simulink model "sysgenConcatenatedFEC"  (Simulink 7.4)
settings: Solver=ode45  SolverMode=SingleTasking  StartTime=0.0  StopTime=5000  RelTol=1e-3
undefined symbols (not defined in the file or in its folder): De, Interleaver, interleaver
libraries: xbsIndex_r4 x119, commchan3 x2, commdigbbndpm3 x2, xbsCopyrightNotice_r4 x1
(part 1 of 2)
settings Model: Creator=alexc  LastModifiedBy=douangp
settings DataIOCC: SignalLoggingName=sigsOut
settings OptimizationCC: BlockReduction=off  BooleanDataType=off  InlineInvariantSignals=on  InitFltsAndDblsToZero=on
settings DebuggingCC: SaveWithParameterizedLinksMsg=none  SignalResolutionControl=TryResolveAllWithWarning  SolverPrmCheckMsg=none  MultiTaskDSMMsg=warning  MultiTaskCondExecSysMsg=none  StrictBusMsg=None
settings HardwareCC: TargetUnknown=on
settings RTWCC: IncludeERTFirstTime=on
settings GRTTargetCC: TargetFcnLib=ansi_tfl_tmw.mat

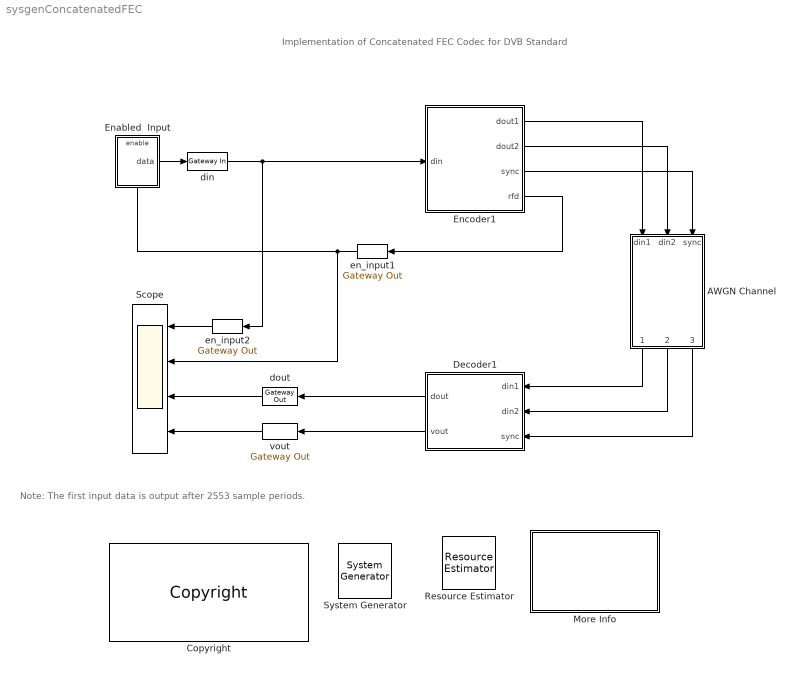
== system sysgenConcatenatedFEC ==
  note: Implementation of Concatenated
      | FEC Codec for DVB Standard
  note: Note: The first input data is output after 2553 sample periods.
  " System Generator" : xbsIndex_r4/ System Generator  Tag=genX  SystemSampleTime=-1  xilinxfamily=virtex6  part=xc6vlx240t  speed=-1  package=ff1156  synthesis_tool=XST  clock_wrapper=Clock Enables  directory=./netlist  testbench=off  simulink_period=1/8  sysclk_period=5  dcm_input_clock_period=100  incr_netlist=off  trim_vbits=Everywhere in SubSystem  dbl_ovrd=According to Block Masks  core_generation=According to Block Masks  run_coregen=off  deprecated_control=off  eval_field=0  block_type=sysgen
      settings: block_version=9.2.00
  AWGN Channel : Subsystem  mask{snr=4}
  Copyright : xbsCopyrightNotice_r4/Copyright  copyrighttext="Copyright (c) 2010  by  Xilinx, Inc. All rights reserved.<br><br>This file contains proprietary, confidential information of Xilinx, Inc., is distributed under licensefrom Xilinx, Inc., and may be used, copied and/or disclosed only pursuant to the terms of a valid licenseagreement with Xilinx, Inc. Xilinx hereby grants you a license to use this file solely for design,simulation, implementation and creation of design files limited to Xilinx devices or technologies. Use with non-Xilinx devices or technologies is expressly prohibited and immediately terminates your license unless covered by a separate agreement.<br><br>Xilinx is providing this design, code, or information \"as-is\" solely for use in developing programs and solutions for Xilinx devices, with no obligation on the part of Xilinx to provide support. By providingthis design, code, or information as one possible implementation of this feature, application or standard,Xilinx is making no representation that this implementation is free from any claims of infringement. Youare responsible for obtaining any rights you may require for your implementation. Xilinx expressly disclaimsany warranty whatsoever with respect to the adequacy of the implementation, including but not limited to anywarranties or representations that this implementation is free from claims of infringement, implied warrantiesof merchantability or fitness for a particular purpose.<br><br>Xilinx products are not intended for use in life support appliances, devices, or systems. Use in such applications is expressly prohibited.<br><br>Any modifications that are made to the Source Code are done at the user's sole risk and will be unsupported.<br><br>This copyright and support notice must be retained as part of this text at all times. (c) Copyright 1995-2010 Xilinx, Inc. All rights reserved."  block_type=copyright
      settings: block_version=10.1.00
      settings: infoedit=|
      | Copyright(C) 2008 by  Xilinx, Inc. All rights reserved.<br>
      | <br>
      | This file contains proprietary, confidential information of Xilinx, Inc., is distributed under license
      | from Xilinx, Inc., and may be used, copied and/or disclosed only pursuant to the terms of a valid license
      | agreement with Xilinx, Inc. Xilinx hereby grants you a license to use this file solely for design,
      | simulation, implementation and creation of design files limited to Xilinx devices or technologies. Use
      | with non-Xilinx devices or technologies is expressly prohibited and immediately terminates your license
      | unless covered by a separate agreement.<br>
      | <br>
      | Xilinx is providing this design, code, or information "as-is" solely for use in developing programs and
      | solutions for Xilinx devices, with no obligation on the part of Xilinx to provide support. By providing
      | this design, code, or information as one possible implementation of this feature, application or standard,
      | Xilinx is making no representation that this implementation is free from any claims of infringement. You
      | are responsible for obtaining any rights you may require for your implementation. Xilinx expressly disclaims
      | any warranty whatsoever with respect to the adequacy of the implementation, including but not limited to any
      | warranties or representations that this implementation is free from claims of infringement, implied warranties
      | of merchantability or fitness for a particular purpose.<br>
      | <br>
      | Xilinx products are not intended for use in life support appliances, devices, or systems. Use in such
      | applications is expressly prohibited.<br>
      | <br>
      | Any modifications that are made to the Source Code are done at the user's sole risk and will be unsupported.<br>
      | <br>
      | This copyright and support notice must be retained as part of this text at all times.
      | (c) Copyright 1995-2008 Xilinx, Inc. All rights reserved.
  Decoder1 : Subsystem
  Enabled  Input : Subsystem  TreatAsAtomicUnit=on
  Encoder1 : Subsystem
  More Info : Subsystem
      mask Display: disp('Double click\n for\n more information.')
  Resource Estimator : xbsIndex_r4/Resource Estimator  Tag=resEstTag  Slices=2727  FFs=2644  BRAMs=8  LUTs=4673  IOBs=27  EBMs=0  TBUFs=0  xl_use_estimator_area=off  est_options=Estimate  xl_estimator_area=[2727 2644 8 4673 27 0 0]  mrp_directory=./sysgenConcatenatedFEC_work  simulink_period=1/8  block_type=resource_estimator
      settings: AttributesFormatString=Resource\nEstimator  block_version=9.2.00
  Scope : Scope  NumInputPorts=4
      settings: TimeRange=5000  YMin=-1~0~-1~0  YMax=0.75~1~1~1  MaxDataPoints=30000
  din : xbsIndex_r4/Gateway In  arith_type="Signed  (2's comp)"  n_bits=8  bin_pt=6  quantization="Round  (unbiased: +/- Inf)"  overflow=Saturate  period=1  dbl_ovrd=off  timing_constraint=None  locs_specified=off  LOCs={}  hdl_port=on  block_type=gatewayin
      settings: infoedit="Gateway in block.  Converts inputs of type Simulink integer, double and fixed point to  Xilinx fixed point type.<P><P>Hardware notes:  In hardware these blocks become top level input ports."  xl_area=[0 0 0 0 8 0 0]  block_version=VER_STRING_GOES_HERE
  dout : xbsIndex_r4/Gateway Out  hdl_port=on  timing_constraint=None  locs_specified=off  LOCs={}  block_type=gatewayout
      settings: infoedit="Gateway out block.  Converts Xilinx fixed point inputs into ouputs of type Simulink integer, double, or fixed point.<P><P>Hardware notes:  In hardware these blocks become top level output ports or are discarded, depending on how they are configured."  xl_area=[0 0 0 0 8 0 0]  block_version=VER_STRING_GOES_HERE
  en_input1 : xbsIndex_r4/Gateway Out  hdl_port=off  timing_constraint=None  locs_specified=off  LOCs={}  block_type=gatewayout
      settings: infoedit="Gateway out block.  Converts Xilinx fixed point inputs into ouputs of type Simulink integer, double, or fixed point.<br><br>Hardware notes:  In hardware these blocks become top level output ports or are discarded, depending on how they are configured."  block_version=11.4
  en_input2 : xbsIndex_r4/Gateway Out  hdl_port=off  timing_constraint=None  locs_specified=off  LOCs={}  block_type=gatewayout
      settings: infoedit="Gateway out block.  Converts Xilinx fixed point inputs into ouputs of type Simulink integer, double, or fixed point.<br><br>Hardware notes:  In hardware these blocks become top level output ports or are discarded, depending on how they are configured."  block_version=11.4
  vout : xbsIndex_r4/Gateway Out  hdl_port=on  timing_constraint=None  locs_specified=off  LOCs={}  block_type=gatewayout
      settings: infoedit="Gateway out block.  Converts Xilinx fixed point inputs into ouputs of type Simulink integer, double, or fixed point.<P><P>Hardware notes:  In hardware these blocks become top level output ports or are discarded, depending on how they are configured."  xl_area=[0 0 0 0 0 0 0]  block_version=VER_STRING_GOES_HERE
  wires:
  Decoder1/1(dout) -> dout/1
  Encoder1/4(rfd) -> en_input1/1
  Enabled  Input/1(data) -> din/1
  din/1 -> en_input2/1, Encoder1/1(din)
  AWGN Channel/1(dout1) -> Decoder1/1(din1)
  AWGN Channel/2(dout2) -> Decoder1/2(din2)
  AWGN Channel/3(sync1) -> Decoder1/3(sync)
  Encoder1/3(sync) -> AWGN Channel/3(sync)
  Encoder1/1(dout1) -> AWGN Channel/1(din1)
  Encoder1/2(dout2) -> AWGN Channel/2(din2)
  Decoder1/2(vout) -> vout/1
  dout/1 -> Scope/3
  vout/1 -> Scope/4
  en_input1/1 -> Scope/2, Enabled  Input/Enable
  en_input2/1 -> Scope/1

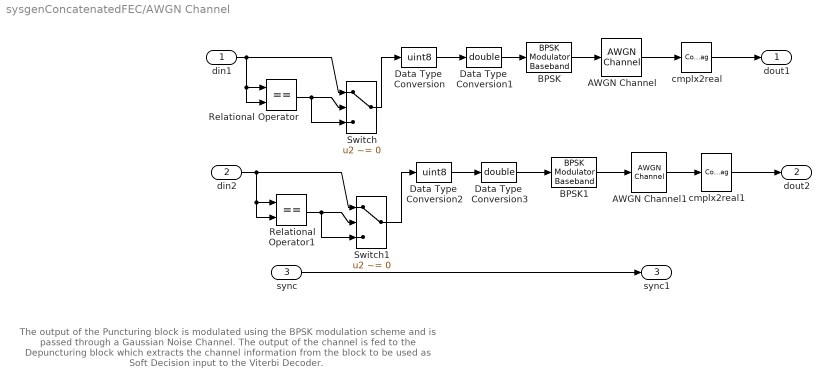
== system sysgenConcatenatedFEC/AWGN Channel ==
  note: The output of the Puncturing block is modulated using the BPSK modulation scheme and  is passed through
      | a Gaussian Noise Channel. The output of the channel is fed to the Depuncturing block which extracts the
      | channel information from the block to be used as Soft Decision input to the Viterbi Decoder.
  din1 : Inport  OutDataType=sfix(16)  OutScaling=2^0
  din2 : Inport  Port=2  OutDataType=sfix(16)  OutScaling=2^0
  sync : Inport  Port=3  OutDataType=sfix(16)  OutScaling=2^0
  AWGN Channel : commchan3/AWGN Channel  SystemSampleTime=-1  seed=54321  noiseMode="Signal to noise ratio  (SNR)"  EbNodB=10  EsNodB=10  SNRdB=snr  bitsPerSym=1  Ps=1  Tsym=1  variance=1
  AWGN Channel1 : commchan3/AWGN Channel  SystemSampleTime=-1  seed=54321  noiseMode="Signal to noise ratio  (SNR)"  EbNodB=10  EsNodB=10  SNRdB=snr  bitsPerSym=1  Ps=1  Tsym=1  variance=1
  BPSK : commdigbbndpm3/BPSK Modulator Baseband  DialogController=commDDGCreate  DialogControllerArgs=DataTag1  SystemSampleTime=-1  Ph=0  outDtype=double  outWordLen=16  outUDDataType=sfix(16)  outFracLenMode=Best precision  outFracLen=15
      link override M-PSK Modulator Baseband: outDtype=double  outFracLenMode=Best precision
  BPSK1 : commdigbbndpm3/BPSK Modulator Baseband  DialogController=commDDGCreate  DialogControllerArgs=DataTag2  SystemSampleTime=-1  Ph=0  outDtype=double  outWordLen=16  outUDDataType=sfix(16)  outFracLenMode=Best precision  outFracLen=15
  Data Type  Conversion : DataTypeConversion  OutDataTypeMode=uint8  OutDataType=sfix(16)  OutScaling=2^0  OutDataTypeStr=uint8  SaturateOnIntegerOverflow=on  RndMeth=Zero
  Data Type  Conversion1 : DataTypeConversion  OutDataTypeMode=double  OutDataType=sfix(16)  OutScaling=2^0  OutDataTypeStr=double  SaturateOnIntegerOverflow=on  RndMeth=Zero
  Data Type  Conversion2 : DataTypeConversion  OutDataTypeMode=uint8  OutDataType=sfix(16)  OutScaling=2^0  OutDataTypeStr=uint8  SaturateOnIntegerOverflow=on  RndMeth=Zero
  Data Type  Conversion3 : DataTypeConversion  OutDataTypeMode=double  OutDataType=sfix(16)  OutScaling=2^0  OutDataTypeStr=double  SaturateOnIntegerOverflow=on  RndMeth=Zero
  Relational Operator : RelationalOperator  Operator===  LogicOutDataTypeMode=boolean  OutDataTypeStr=boolean
  Relational Operator1 : RelationalOperator  Operator===  LogicOutDataTypeMode=boolean  OutDataTypeStr=boolean
  Switch : Switch  Criteria=u2 ~= 0
  Switch1 : Switch  Criteria=u2 ~= 0
  cmplx2real : ComplexToRealImag  Output=Real
  cmplx2real1 : ComplexToRealImag  Output=Real
  dout1 : Outport  OutDataType=sfix(16)  OutScaling=2^0
  dout2 : Outport  Port=2  OutDataType=sfix(16)  OutScaling=2^0
  sync1 : Outport  Port=3  OutDataType=sfix(16)  OutScaling=2^0
  wires:
  BPSK/1 -> AWGN Channel/1
  BPSK1/1 -> AWGN Channel1/1
  AWGN Channel/1 -> cmplx2real/1
  AWGN Channel1/1 -> cmplx2real1/1
  cmplx2real/1 -> dout1/1
  cmplx2real1/1 -> dout2/1
  sync/1 -> sync1/1
  Data Type  Conversion3/1 -> BPSK1/1
  Data Type  Conversion1/1 -> BPSK/1
  Data Type  Conversion/1 -> Data Type  Conversion1/1
  Data Type  Conversion2/1 -> Data Type  Conversion3/1
  din1/1 -> Relational Operator/1, Relational Operator/2, Switch/1
  Relational Operator/1 -> Switch/2, Switch/3
  Switch/1 -> Data Type  Conversion/1
  din2/1 -> Relational Operator1/1, Relational Operator1/2, Switch1/1
  Relational Operator1/1 -> Switch1/2, Switch1/3
  Switch1/1 -> Data Type  Conversion2/1

== system sysgenConcatenatedFEC/Decoder1 ==
  note: Depuncturing
  note: Inner
      | Decoder
  note: Convolutional
      | Deinterleaver
  note: Outer
      | Decoder
  note: Concatenated Decoder
  din1 : Inport  OutDataType=sfix(16)  OutScaling=2^0
  din2 : Inport  Port=2  OutDataType=sfix(16)  OutScaling=2^0
  sync : Inport  Port=3  OutDataType=sfix(16)  OutScaling=2^0
  cvdeint : Subsystem
  depunc : Subsystem
  rsdec : Subsystem
  vitdec : Subsystem
  dout : Outport  OutDataType=sfix(16)  OutScaling=2^0
  vout : Outport  Port=2  OutDataType=sfix(16)  OutScaling=2^0
  wires:
  rsdec/2(data1) -> vout/1
  rsdec/1(data) -> dout/1
  sync/1 -> depunc/3(sync)
  din2/1 -> depunc/2(din2)
  din1/1 -> depunc/1(din1)
  cvdeint/2(vout) -> rsdec/2(vin)
  vitdec/2(vout) -> cvdeint/2(vin)
  depunc/3(vin) -> vitdec/3(vin)
  cvdeint/1(dout) -> rsdec/1(din)
  vitdec/1(dout) -> cvdeint/1(din)
  depunc/2(dout2) -> vitdec/2(din2)
  depunc/1(dout1) -> vitdec/1(din1)

== system sysgenConcatenatedFEC/Enabled  Input ==
  note: The input to the concatenated coder is a sine wave which is enabled using the RFD (Ready for Data)
      | output of the Outer Encoder.
  Enable : EnablePort  PropagateVarSize=During execution
  Sine Wave : Sin  SineType=Sample based  Amplitude=1  Bias=0  Frequency=1  Phase=0  Samples=60  SampleTime=1  Offset=0
  data : Outport  OutDataType=sfix(16)  OutScaling=2^0
  wires:
  Sine Wave/1 -> data/1

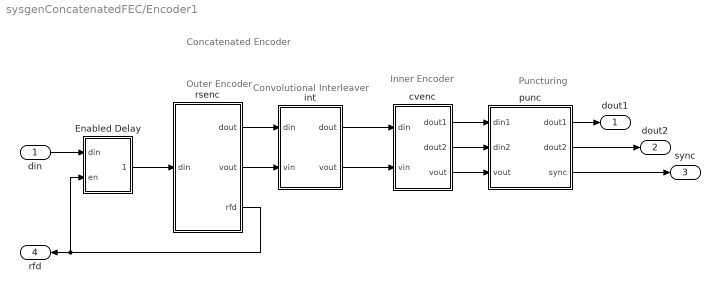
== system sysgenConcatenatedFEC/Encoder1 ==
  note: Outer
      | Encoder
  note: Convolutional
      | Interleaver
  note: Inner
      | Encoder
  note: Puncturing
  note: Concatenated Encoder
  din : Inport  OutDataType=sfix(16)  OutScaling=2^0
  Enabled Delay : Subsystem
  cvenc : Subsystem
  int : Subsystem
  punc : Subsystem
  rsenc : Subsystem
  dout1 : Outport  OutDataType=sfix(16)  OutScaling=2^0
  dout2 : Outport  Port=2  OutDataType=sfix(16)  OutScaling=2^0
  sync : Outport  Port=3  OutDataType=sfix(16)  OutScaling=2^0
  rfd : Outport  Port=4  OutDataType=sfix(16)  OutScaling=2^0
  wires:
  Enabled Delay/1(dout) -> rsenc/1(din)
  din/1 -> Enabled Delay/1(din)
  rsenc/1(dout) -> int/1(din)
  int/1(dout) -> cvenc/1(din)
  rsenc/2(vout) -> int/2(vin)
  int/2(vout) -> cvenc/2(vin)
  cvenc/3(vout) -> punc/3(vout)
  cvenc/2(dout2) -> punc/2(din2)
  cvenc/1(dout1) -> punc/1(din1)
  punc/3(sync) -> sync/1
  punc/2(dout2) -> dout2/1
  punc/1(dout1) -> dout1/1
  rsenc/3(rfd) -> Enabled Delay/2(en), rfd/1

== system sysgenConcatenatedFEC/More Info ==
  note: This design demonstrates a concatenated forward error correction scheme using the
      |  blocks provided in the Xilinx Communication library. The scheme is implemented
      | according to the specifications provided in the European Telecommunication Standard
      | (ETS 300 421) for Digital Video Broadcasting.
  note: Implementation of Concatenated FEC Codec for DVB Standard

== system sysgenConcatenatedFEC/Decoder1/cvdeint ==
  note: The Convolutional Deinterleaver specified in the standard is implemented by selecting Deinterleaver mode in the
      | Interleaver Deinterleaver block in the Xilinx Communication library. The Deinterleaver has 12 branches with the
      | constant difference between branch lengths being 17 shift registers. The convolutional deinterleaving is based on
      | the Forney type architecture. The Deinterleaver block synchronizes its output to the first valid data received at the input.
      | The Delay block at the input of the deinterleaver is used for pipelining the design.
      |
      | A single pulse is required at the "fd" (First Data) input and it has to be lined up with the "nd" (New Data) signal.
      | To accomplish this,  a simple single-shot circuit is used (Rising Edge Detector) to detect a low-to-high transition from "vin".
  din : Inport  OutDataType=sfix(16)  OutScaling=2^0
  vin : Inport  Port=2  OutDataType=sfix(16)  OutScaling=2^0
  Delay : xbsIndex_r4/Delay  en=off  latency=1  dbl_ovrd=off  reg_retiming=off  block_type=delay
      settings: infoedit="Delay line having  configurable length.<P><P>Hardware notes: A delay line is a chain, each link of which is an SRL16 followed by a flip-flop. If register retiming is enabled, the delay line is a chain of flip-flops."  xl_area=[0, 0, 0, 0, 0, 0, 0]  block_version=VER_STRING_GOES_HERE
  Delay1 : xbsIndex_r4/Delay  en=off  latency=1  dbl_ovrd=off  reg_retiming=off  block_type=delay
      settings: infoedit="Delay line having  configurable length.<P><P>Hardware notes: A delay line is a chain, each link of which is an SRL16 followed by a flip-flop. If register retiming is enabled, the delay line is a chain of flip-flops."  xl_area=[0, 0, 0, 0, 0, 0, 0]  block_version=VER_STRING_GOES_HERE
  "Interleaver/De-interleaver 6.0 " : xbsIndex_r4/Interleaver//De-interleaver 6.0   memory_style=Automatic  symbol_width=8  sid_type=Forney  mode=Deinterleaver  symbol_memory=Internal  number_of_branches=12  architecture=ROM_based  number_of_configurations=1  branch_length_constant=17  branch_length_coe_file_name='no_coe_file_loaded'  branch_length_type=constant_difference_between_consecutive_branches  number_of_rows_constant_value=15  row_port_width=4  minimum_rows=15  number_of_rows_selectable_value=4  number_of_rows=constant  number_of_columns_constant_value=15  col_port_width=4  minimum_columns=15  number_of_columns_selectable_value=4  number_of_columns=constant  row_permutations=None  column_permutations=None  coe_file='no_coe_file_loaded'  block_size_constant_value=225  block_size_port_width=8  block_size_type=rows_columns  row_valid=off  block_size_valid=off  ce=off  rfd=off  row_sel_valid=off  block_start=off  sclr=off  rffd=off  col_valid=off  block_end=off  ndo=off  fdo=off  col_sel_valid=off  nd=on  rdy=on  pipelining=minimum  ip_name=Interleaver/De-interleaver  ip_version=6.0  dsptool_ready=true  ipcore_usecache=true  ipcore_useipmodelcache=true  wrapper_available=true  port_translation_map={ 'ce' => 'en', 'sclr' => 'rst'}  structural_sim=false  ipcore_verbose=false  ipcore_do_not_force_period=true  block_type=sid_v6_0
      settings: infoedit=Forney Information : The Forney type is composed of a user-defined number of delay-line shift registers. The length of each of the delay-line shift registers can be specified using a COE file, or by setting the difference in the length of consecutive delay line shift registers to a fixed, user-defined value. <br> Rectangular Information : The Rectangular Block type is composed of a rectangular array of memory elements, where the number of rows and columns in the array is user-defined. The number of rows and columns can be constant or run-time configurable. The elements are written to row-wise, and read out column-wise, or vice versa, depending on which mode is selected. This type supports user-defined inter-row and inter-column permutations. It also supports pruning - cases where the block size is less than the product of the number of rows and columns.  block_version=12.1
  Rising Edge Detector1 : Subsystem
  dout : Outport  OutDataType=sfix(16)  OutScaling=2^0
  vout : Outport  Port=2  OutDataType=sfix(16)  OutScaling=2^0
  wires:
  "Interleaver/De-interleaver 6.0 "/2 -> vout/1
  vin/1 -> Rising Edge Detector1/1(Din), Delay1/1
  din/1 -> Delay/1
  "Interleaver/De-interleaver 6.0 "/1 -> dout/1
  Delay/1 -> "Interleaver/De-interleaver 6.0 "/1
  Delay1/1 -> "Interleaver/De-interleaver 6.0 "/2
  Rising Edge Detector1/1(Dout) -> "Interleaver/De-interleaver 6.0 "/3

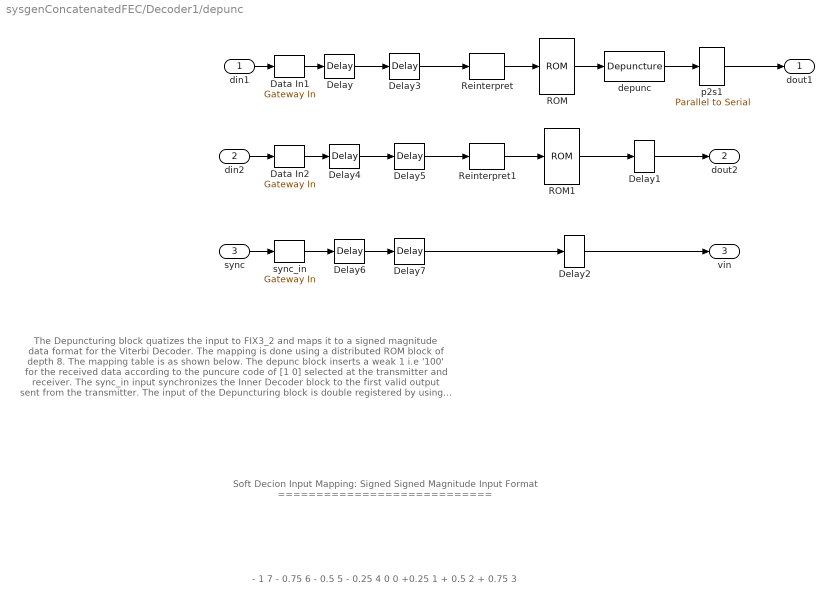
== system sysgenConcatenatedFEC/Decoder1/depunc ==
  note: Soft Decion Input Mapping:
      |
      | Signed            Signed Magnitude
      | Input                Format
      | ============================
  note: - 1                                7
      | - 0.75                                 6
      | - 0.5                                  5
      | - 0.25                                 4
      | 0                                0
      | +0.25                                 1
      | + 0.5                                  2
      | + 0.75                                 3
  note: The Depuncturing block quatizes the input to FIX3_2 and maps it to a signed magnitude data format for
      | the Viterbi Decoder. The mapping is done using a distributed ROM block of depth 8. The mapping table is
      | as shown below. The depunc block inserts a weak 1 i.e '100' for the received data according to the puncure
      | code of  [1 0] selected at the transmitter and receiver. The sync_in input synchronizes the Inner Decoder block
      | to the first valid output sent from the transmitter. The input of the Depuncturing block is double registered by using
      | the delay blocks.
  din1 : Inport  OutDataType=sfix(16)  OutScaling=2^0
  din2 : Inport  Port=2  OutDataType=sfix(16)  OutScaling=2^0
  sync : Inport  Port=3  OutDataType=sfix(16)  OutScaling=2^0
  Data In1 : xbsIndex_r4/Gateway In  arith_type="Signed  (2's comp)"  n_bits=3  bin_pt=2  quantization="Round  (unbiased: +/- Inf)"  overflow=Saturate  period=1/4  dbl_ovrd=off  timing_constraint=None  locs_specified=off  LOCs={}  hdl_port=on  block_type=gatewayin
      settings: infoedit="Gateway in block.  Converts inputs of type Simulink integer, double and fixed point to  Xilinx fixed point type.<P><P>Hardware notes:  In hardware these blocks become top level input ports."  xl_area=[0 0 0 0 3 0 0]  block_version=VER_STRING_GOES_HERE
  Data In2 : xbsIndex_r4/Gateway In  arith_type="Signed  (2's comp)"  n_bits=3  bin_pt=2  quantization="Round  (unbiased: +/- Inf)"  overflow=Saturate  period=1/8  dbl_ovrd=off  timing_constraint=None  locs_specified=off  LOCs={}  hdl_port=on  block_type=gatewayin
      settings: infoedit="Gateway in block.  Converts inputs of type Simulink integer, double and fixed point to  Xilinx fixed point type.<P><P>Hardware notes:  In hardware these blocks become top level input ports."  xl_area=[0 0 0 0 3 0 0]  block_version=VER_STRING_GOES_HERE
  Delay{,3..7} (6 alike) : xbsIndex_r4/Delay  en=off  latency=1  dbl_ovrd=off  reg_retiming=off  block_type=delay
      Delay settings: infoedit="Delay line having  configurable length.<P><P>Hardware notes: A delay line is a chain, each link of which is an SRL16 followed by a flip-flop. If register retiming is enabled, the delay line is a chain of flip-flops."  xl_area=[2 3 0 0 0 0 0]  block_version=VER_STRING_GOES_HERE
      Delay3 settings: infoedit="Delay line having  configurable length.<P><P>Hardware notes: A delay line is a chain, each link of which is an SRL16 followed by a flip-flop. If register retiming is enabled, the delay line is a chain of flip-flops."  xl_area=[2 3 0 0 0 0 0]  block_version=VER_STRING_GOES_HERE
      Delay4 settings: infoedit="Delay line having  configurable length.<P><P>Hardware notes: A delay line is a chain, each link of which is an SRL16 followed by a flip-flop. If register retiming is enabled, the delay line is a chain of flip-flops."  xl_area=[2 3 0 0 0 0 0]  block_version=VER_STRING_GOES_HERE
      Delay5 settings: infoedit="Delay line having  configurable length.<P><P>Hardware notes: A delay line is a chain, each link of which is an SRL16 followed by a flip-flop. If register retiming is enabled, the delay line is a chain of flip-flops."  xl_area=[2 3 0 0 0 0 0]  block_version=VER_STRING_GOES_HERE
      Delay6 settings: infoedit="Delay line having  configurable length.<P><P>Hardware notes: A delay line is a chain, each link of which is an SRL16 followed by a flip-flop. If register retiming is enabled, the delay line is a chain of flip-flops."  xl_area=[1 1 0 0 0 0 0]  block_version=VER_STRING_GOES_HERE
      Delay7 settings: infoedit="Delay line having  configurable length.<P><P>Hardware notes: A delay line is a chain, each link of which is an SRL16 followed by a flip-flop. If register retiming is enabled, the delay line is a chain of flip-flops."  xl_area=[1 1 0 0 0 0 0]  block_version=VER_STRING_GOES_HERE
  Delay1 : xbsIndex_r4/Delay  en=off  latency=6  dbl_ovrd=off  reg_retiming=off  block_type=delay
      settings: infoedit="Delay line having  configurable length.<P><P>Hardware notes: A delay line is a chain, each link of which is an SRL16 followed by a flip-flop. If register retiming is enabled, the delay line is a chain of flip-flops."  xl_area=[2 3 0 3 0 0 0]  block_version=VER_STRING_GOES_HERE
  Delay2 : xbsIndex_r4/Delay  en=off  latency=6  dbl_ovrd=off  reg_retiming=off  block_type=delay
      settings: infoedit="Delay line having  configurable length.<P><P>Hardware notes: A delay line is a chain, each link of which is an SRL16 followed by a flip-flop. If register retiming is enabled, the delay line is a chain of flip-flops."  xl_area=[1 1 0 1 0 0 0]  block_version=VER_STRING_GOES_HERE
  ROM : xbsIndex_r4/ROM  depth=8  initVector="[ 0  1 2 3 7 6 5 4]"  distributed_mem=Distributed memory  rst=off  init_reg=0  en=off  latency=0  arith_type=Unsigned  n_bits=3  bin_pt=0  dbl_ovrd=off  optimize=Area  use_rpm=off  block_type=sprom
      settings: xl_area=[2 0 0 3 0 0 0]  block_version=VER_STRING_GOES_HERE
  ROM1 : xbsIndex_r4/ROM  depth=8  initVector="[ 0  1 2 3 7 6 5 4]"  distributed_mem=Distributed memory  rst=off  init_reg=0  en=off  latency=0  arith_type=Unsigned  n_bits=3  bin_pt=0  dbl_ovrd=off  optimize=Area  use_rpm=off  block_type=sprom
      settings: xl_area=[2 0 0 3 0 0 0]  block_version=VER_STRING_GOES_HERE
  Reinterpret : xbsIndex_r4/Reinterpret  force_arith_type=on  arith_type=Unsigned  force_bin_pt=on  bin_pt=0  block_type=cast
      settings: infoedit="Changes type of samples without altering their binary representation.<P><P>Hardware notes: In hardware this block costs nothing.<P><P>Example:  Suppose the input is 6 bits wide, signed, with 2 fractional bits, and the output is forced to unsigned with 0 fractional bits.  Then an input of -2.0 (1110.00 in binary 2's complement) becomes an output of 56 (111000 in binary)."  block_version=VER_STRING_GOES_HERE
  Reinterpret1 : xbsIndex_r4/Reinterpret  force_arith_type=on  arith_type=Unsigned  force_bin_pt=on  bin_pt=0  block_type=cast
      settings: infoedit="Changes type of samples without altering their binary representation.<P><P>Hardware notes: In hardware this block costs nothing.<P><P>Example:  Suppose the input is 6 bits wide, signed, with 2 fractional bits, and the output is forced to unsigned with 0 fractional bits.  Then an input of -2.0 (1110.00 in binary 2's complement) becomes an output of 56 (111000 in binary)."  block_version=VER_STRING_GOES_HERE
  depunc : xbsIndex_r4/Depuncture  insert_char=[1 0]  insert_string='100'  dbl_ovrd=off  block_type=insert
      settings: infoedit="Depunctures convolutional codes.  Reads values from the input port, then inserts symbols at the locations specified by zeros in the puncture code, and presents the results at the output port. <P><P>Hardware notes: In hardware this block costs nothing."  block_version=VER_STRING_GOES_HERE
  p2s1 : xbsIndex_r4/Parallel to Serial  output_order=Least Significant Word First  arith_type=Unsigned  output_bits=3  bin_pt=0  en=off  latency=0  dbl_ovrd=off  block_type=p2s
      settings: infoedit=Each sample presented at the input becomes several samples presented serially at the output.  xl_area=[6 7 0 6 0 0 0]  block_version=VER_STRING_GOES_HERE
  sync_in : xbsIndex_r4/Gateway In  arith_type=Boolean  n_bits=1  bin_pt=0  quantization="Round  (unbiased: +/- Inf)"  overflow=Saturate  period=1/8  dbl_ovrd=off  timing_constraint=None  locs_specified=off  LOCs={}  hdl_port=on  block_type=gatewayin
      settings: infoedit="Gateway in block.  Converts inputs of type Simulink integer, double and fixed point to  Xilinx fixed point type.<P><P>Hardware notes:  In hardware these blocks become top level input ports."  xl_area=[0 0 0 0 1 0 0]  block_version=VER_STRING_GOES_HERE
  dout1 : Outport  OutDataType=sfix(16)  OutScaling=2^0
  dout2 : Outport  Port=2  OutDataType=sfix(16)  OutScaling=2^0
  vin : Outport  Port=3  OutDataType=sfix(16)  OutScaling=2^0
  wires:
  Delay7/1 -> Delay2/1
  sync_in/1 -> Delay6/1
  Delay6/1 -> Delay7/1
  Delay5/1 -> Reinterpret1/1
  Data In2/1 -> Delay4/1
  Delay4/1 -> Delay5/1
  Data In1/1 -> Delay/1
  Delay3/1 -> Reinterpret/1
  Delay/1 -> Delay3/1
  Delay2/1 -> vin/1
  Delay1/1 -> dout2/1
  p2s1/1 -> dout1/1
  ROM/1 -> depunc/1
  depunc/1 -> p2s1/1
  sync/1 -> sync_in/1
  Reinterpret1/1 -> ROM1/1
  ROM1/1 -> Delay1/1
  Reinterpret/1 -> ROM/1
  din2/1 -> Data In2/1
  din1/1 -> Data In1/1

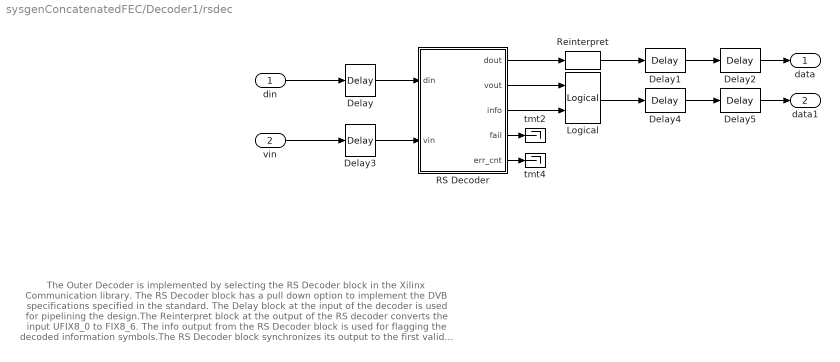
== system sysgenConcatenatedFEC/Decoder1/rsdec ==
  note: The Outer Decoder is implemented by selecting  the RS Decoder block in the Xilinx Communication library. The
      | RS Decoder block has a pull down option to implement the DVB specifications specified in the standard. The Delay
      | block at the input of the decoder is used for pipelining the design.The Reinterpret block at the output of the RS
      | decoder converts the input UFIX8_0 to FIX8_6. The info output from the RS Decoder block is used for flagging the
      | decoded information symbols.The RS Decoder block synchronizes its output to the first valid data received at the
      | input. ThE RS decoder also has fail and err_cnt outputs which flag failure in decodng a particular data frame and
      | the number of errors corrected by the RS decoder.
  din : Inport  OutDataType=sfix(16)  OutScaling=2^0
  vin : Inport  Port=2  OutDataType=sfix(16)  OutScaling=2^0
  Delay{,1..5} (6 alike) : xbsIndex_r4/Delay  en=off  latency=1  dbl_ovrd=off  reg_retiming=off  block_type=delay
      settings: infoedit="Delay line having  configurable length.<P><P>Hardware notes: A delay line is a chain, each link of which is an SRL16 followed by a flip-flop. If register retiming is enabled, the delay line is a chain of flip-flops."  xl_area=[0, 0, 0, 0, 0, 0, 0]  block_version=VER_STRING_GOES_HERE
  Logical : xbsIndex_r4/Logical  logical_function=AND  inputs=2  en=off  latency=0  precision=Full  arith_type=Unsigned  n_bits=8  bin_pt=2  align_bp=on  dbl_ovrd=off  block_type=logical
      settings: block_version=VER_STRING_GOES_HERE
  RS Decoder : Subsystem
      settings: CopyFcn=set_param(gcb, 'LinkStatus', 'none');
  Reinterpret : xbsIndex_r4/Reinterpret  force_arith_type=on  arith_type="Signed  (2's comp)"  force_bin_pt=on  bin_pt=6  block_type=cast
      settings: infoedit="Changes type of samples without altering their binary representation.<P><P>Hardware notes: In hardware this block costs nothing.<P><P>Example:  Suppose the input is 6 bits wide, signed, with 2 fractional bits, and the output is forced to unsigned with 0 fractional bits.  Then an input of -2.0 (1110.00 in binary 2's complement) becomes an output of 56 (111000 in binary)."  block_version=VER_STRING_GOES_HERE
  tmt2 : Terminator
  tmt4 : Terminator
  data : Outport  OutDataType=sfix(16)  OutScaling=2^0
  data1 : Outport  Port=2  OutDataType=sfix(16)  OutScaling=2^0
  wires:
  Logical/1 -> Delay4/1
  Delay5/1 -> data1/1
  Delay4/1 -> Delay5/1
  RS Decoder/1(dout) -> Reinterpret/1
  Delay/1 -> RS Decoder/1(din)
  vin/1 -> Delay3/1
  Delay3/1 -> RS Decoder/2(vin)
  RS Decoder/5(err_cnt) -> tmt4/1
  RS Decoder/2(vout) -> Logical/1
  Delay2/1 -> data/1
  Delay1/1 -> Delay2/1
  RS Decoder/3(info) -> Logical/2
  din/1 -> Delay/1
  RS Decoder/4(fail) -> tmt2/1
  Reinterpret/1 -> Delay1/1

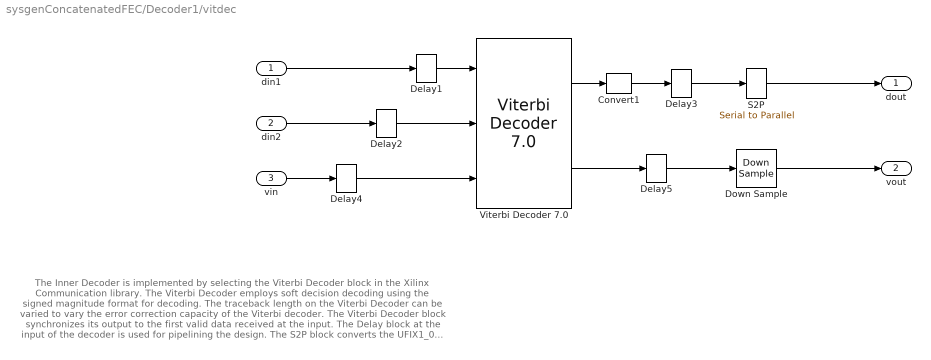
== system sysgenConcatenatedFEC/Decoder1/vitdec ==
  note: The Inner Decoder is implemented by selecting  the Viterbi Decoder block in the Xilinx Communication library.
      | The Viterbi Decoder employs soft decision decoding using the signed magnitude format for decoding. The traceback
      | length on the Viterbi Decoder can be varied to vary the error correction capacity of the Viterbi decoder. The Viterbi
      | Decoder block synchronizes its output to the first valid data received at the input. The Delay block at the input of the
      | decoder is used for pipelining the design. The S2P block converts the UFIX1_0 input to UFIX8_0 for the
      | Deinterleaver block.
  din1 : Inport  OutDataType=sfix(16)  OutScaling=2^0
  din2 : Inport  Port=2  OutDataType=sfix(16)  OutScaling=2^0
  vin : Inport  Port=3  OutDataType=sfix(16)  OutScaling=2^0
  Convert1 : xbsIndex_r4/Convert  arith_type=Unsigned  n_bits=1  bin_pt=0  quantization=Truncate  overflow=Wrap  en=off  latency=0  dbl_ovrd=off  pipeline=off  block_type=convert
      settings: block_version=11.4
  Delay{1..5} (5 alike) : xbsIndex_r4/Delay  en=off  latency=1  dbl_ovrd=off  reg_retiming=off  block_type=delay
      settings: infoedit="Delay line having  configurable length.<P><P>Hardware notes: A delay line is a chain, each link of which is an SRL16 followed by a flip-flop. If register retiming is enabled, the delay line is a chain of flip-flops."  xl_area=[0, 0, 0, 0, 0, 0, 0]  block_version=VER_STRING_GOES_HERE
  Down Sample : xbsIndex_r4/Down Sample  sample_ratio=8  sample_phase="Last Value of Frame  (most efficient)"  en=off  latency=1  dbl_ovrd=off  block_type=dsamp
      settings: xl_area=[0, 0, 0, 0, 0, 0, 0]  block_version=VER_STRING_GOES_HERE
  S2P : xbsIndex_r4/Serial to Parallel  input_order=Least Significant Word First  arith_type=Unsigned  output_bits=8  bin_pt=0  en=off  latency=1  dbl_ovrd=off  block_type=s2p
      settings: infoedit=Groups of samples presented serially at the input become single samples presented at the output.  xl_area=[0, 0, 0, 0, 0, 0, 0]  block_version=VER_STRING_GOES_HERE
  "Viterbi Decoder 7.0 " : xbsIndex_r4/Viterbi Decoder 7.0   channels=1  viterbi_type=Standard  reduced_latency=off  constraint_length=7  traceback_length=96  architecture=Parallel  best_state=off  best_state_width=3  soft_width=3  coding=Soft_Coding  data_format=Signed_Magnitude  output_rate0=2  convolution_code_0_radix=Binary  convolution0_code0='1001111'  convolution0_code1='1010111'  convolution0_code2='0'  convolution0_code3='0'  convolution0_code4='0'  convolution0_code5='0'  convolution0_code6='0'  output_rate1=2  convolution_code_1_radix=Binary  convolution1_code0='1111001'  convolution1_code1='1011011'  convolution1_code2='0'  convolution1_code3='0'  convolution1_code4='0'  convolution1_code5='0'  convolution1_code6='0'  trellis_initialization=None  maximum_direct=96  direct_traceback=None  puncturing=None  ber_symbol_count=off  number_of_ber_symbols=300  synchronization=off  dynamic_thresholds=off  ber_thresh=600  norm_thresh=250  ce=off  rdy=off  synchronous_clear=off  norm=off  block_valid=on  ip_name=Viterbi Decoder  ip_version=7.0  dsptool_ready=false  ipcore_usecache=true  ipcore_useipmodelcache=true  wrapper_available=true  port_translation_map={ 'ce' => 'en', 'sclr' => 'rst'}  structural_sim=false  block_type=viterbi_v7_0
      settings: block_version=11.4
  dout : Outport  OutDataType=sfix(16)  OutScaling=2^0
  vout : Outport  Port=2  OutDataType=sfix(16)  OutScaling=2^0
  wires:
  Convert1/1 -> Delay3/1
  "Viterbi Decoder 7.0 "/2 -> Delay5/1
  Down Sample/1 -> vout/1
  Delay5/1 -> Down Sample/1
  Delay4/1 -> "Viterbi Decoder 7.0 "/3
  vin/1 -> Delay4/1
  Delay3/1 -> S2P/1
  Delay2/1 -> "Viterbi Decoder 7.0 "/2
  Delay1/1 -> "Viterbi Decoder 7.0 "/1
  din2/1 -> Delay2/1
  S2P/1 -> dout/1
  din1/1 -> Delay1/1
  "Viterbi Decoder 7.0 "/1 -> Convert1/1

== system sysgenConcatenatedFEC/Encoder1/Enabled Delay ==
  note: The delay blocks are used for double registering the I/Os on the FPGA.
  din : Inport  OutDataType=sfix(16)  OutScaling=2^0
  en : Inport  Port=2  OutDataType=sfix(16)  OutScaling=2^0
  Convert : xbsIndex_r4/Convert  arith_type=Boolean  n_bits=8  bin_pt=6  quantization=Truncate  overflow=Wrap  en=off  latency=0  dbl_ovrd=off  pipeline=off  block_type=convert
      settings: infoedit=The input is presented at the output after quantization and overflow effects.<P><P>Hardware notes: Additional hardware is used when rounding or saturation is selected and output width is less than the input width.  xl_area=[0 0 0 0 0 0 0]  block_version=VER_STRING_GOES_HERE
  Delay : xbsIndex_r4/Delay  en=on  latency=1  dbl_ovrd=off  reg_retiming=off  block_type=delay
      settings: infoedit="Delay line having  configurable length.<P><P>Hardware notes: A delay line is a chain, each link of which is an SRL16 followed by a flip-flop. If register retiming is enabled, the delay line is a chain of flip-flops."  xl_area=[4 8 0 0 0 0 0]  block_version=VER_STRING_GOES_HERE
  Delay1 : xbsIndex_r4/Delay  en=on  latency=1  dbl_ovrd=off  reg_retiming=off  block_type=delay
      settings: infoedit="Delay line having  configurable length.<P><P>Hardware notes: A delay line is a chain, each link of which is an SRL16 followed by a flip-flop. If register retiming is enabled, the delay line is a chain of flip-flops."  xl_area=[4 8 0 0 0 0 0]  block_version=VER_STRING_GOES_HERE
  dout : Outport  OutDataType=sfix(16)  OutScaling=2^0
  wires:
  Convert/1 -> Delay1/2, Delay/2
  en/1 -> Convert/1
  din/1 -> Delay/1
  Delay1/1 -> dout/1
  Delay/1 -> Delay1/1

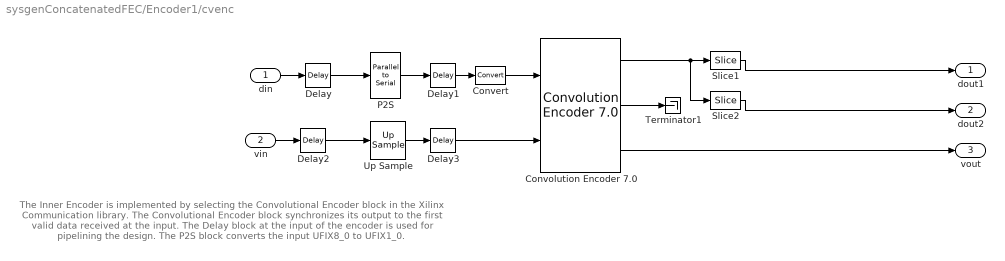
== system sysgenConcatenatedFEC/Encoder1/cvenc ==
  note: The Inner Encoder is implemented by selecting  the Convolutional Encoder block in the Xilinx Communication library.
      | The Convolutional Encoder block synchronizes its output to the first valid data received at the input. The Delay block at
      |  the input of the encoder is used for pipelining the design. The P2S block converts the input UFIX8_0 to UFIX1_0.
  din : Inport  OutDataType=sfix(16)  OutScaling=2^0
  vin : Inport  Port=2  OutDataType=sfix(16)  OutScaling=2^0
  Convert : xbsIndex_r4/Convert  arith_type=Boolean  n_bits=16  bin_pt=14  quantization=Truncate  overflow=Wrap  en=off  latency=0  dbl_ovrd=off  pipeline=off  block_type=convert
      settings: block_version=11.4
  "Convolution Encoder 7.0 " : xbsIndex_r4/Convolution Encoder 7.0   input_rate=1  output_rate=2  punctured=off  dual_output=off  puncture_code0='0'  puncture_code1='0'  constraint_length=7  convolution_code0='1001111'  convolution_code1='1010111'  convolution_code2='0000011'  convolution_code3='0000011'  convolution_code4='0000011'  convolution_code5='0000011'  convolution_code6='0000011'  nd=on  rfd=on  fd_in=off  rffd=off  rdy=on  synchronous_clear=off  ce=off  ip_name=Convolution Encoder  ip_version=7.0  dsptool_ready=false  ipcore_usecache=true  ipcore_useipmodelcache=true  wrapper_available=true  port_translation_map={ 'ce' => 'en', 'sclr' => 'rst'}  structural_sim=true  ipcore_do_not_force_period=true  block_type=convolution_v7_0
      settings: block_version=11.4
  Delay{,1..3} (4 alike) : xbsIndex_r4/Delay  en=off  latency=1  dbl_ovrd=off  reg_retiming=off  block_type=delay
      settings: infoedit="Delay line having  configurable length.<P><P>Hardware notes: A delay line is a chain, each link of which is an SRL16 followed by a flip-flop. If register retiming is enabled, the delay line is a chain of flip-flops."  xl_area=[0, 0, 0, 0, 0, 0, 0]  block_version=VER_STRING_GOES_HERE
  P2S : xbsIndex_r4/Parallel to Serial  output_order=Least Significant Word First  arith_type=Unsigned  output_bits=1  bin_pt=0  en=off  latency=0  dbl_ovrd=off  block_type=p2s
      settings: infoedit=Each sample presented at the input becomes several samples presented serially at the output.  xl_area=[0, 0, 0, 0, 0, 0, 0]  block_version=VER_STRING_GOES_HERE
  Slice1 : xbsIndex_r4/Slice  nbits=1  boolean_output=off  mode=Lower Bit Location + Width  bit1=0  base1=MSB of Input  bit0=0  base0=LSB of Input  dbl_ovrd=off  block_type=slice
  Slice2 : xbsIndex_r4/Slice  nbits=1  boolean_output=off  mode=Upper Bit Location + Width  bit1=0  base1=MSB of Input  bit0=0  base0=LSB of Input  dbl_ovrd=off  block_type=slice
  Terminator1 : Terminator
  Up Sample : xbsIndex_r4/Up Sample  sample_ratio=8  copy_samples=on  en=off  latency=0  dbl_ovrd=off  block_type=usamp
      settings: infoedit="Up samples input data.  Inserted values  can be zeros or copies of the most recent input sample.<P><P>Hardware notes: No hardware is needed if inserted values are copies of the input sample; otherwise, a mux and single bit flip-flop are used."  xl_area=[0, 0, 0, 0, 0, 0, 0]  block_version=VER_STRING_GOES_HERE
  dout1 : Outport  OutDataType=sfix(16)  OutScaling=2^0
  dout2 : Outport  Port=2  OutDataType=sfix(16)  OutScaling=2^0
  vout : Outport  Port=3  OutDataType=sfix(16)  OutScaling=2^0
  wires:
  Slice2/1 -> dout2/1
  Slice1/1 -> dout1/1
  Convert/1 -> "Convolution Encoder 7.0 "/1
  "Convolution Encoder 7.0 "/2 -> Terminator1/1
  "Convolution Encoder 7.0 "/1 -> Slice2/1, Slice1/1
  "Convolution Encoder 7.0 "/3 -> vout/1
  Delay3/1 -> "Convolution Encoder 7.0 "/2
  Up Sample/1 -> Delay3/1
  Delay2/1 -> Up Sample/1
  vin/1 -> Delay2/1
  Delay1/1 -> Convert/1
  Delay/1 -> P2S/1
  din/1 -> Delay/1
  P2S/1 -> Delay1/1

== system sysgenConcatenatedFEC/Encoder1/int ==
  note: The Convolutional Interleaver specified in the standard is implemented by selecting Interleaver mode in the
      | Interleaver Deinterleaver block in the Xilinx Communication library. The Interleaver has 12 branches with the
      | constant difference between branch lengths being 17 shift registers. The convolutional interleaving is based on
      | the Forney type architecture. The Interleaver block synchronizes its output to the first valid data received at the input.
      | The Delay block at the input of the interleaver is used for pipelining the design.
      |
      | A single pulse is required at the "fd" (First Data) input and it has to be lined up with the "nd" (New Data) signal.
      | To accomplish this,  a simple single-shot circuit is used (Rising Edge Detector) to detect a low-to-high transition from "vin".
  din : Inport  OutDataType=sfix(16)  OutScaling=2^0
  vin : Inport  Port=2  OutDataType=sfix(16)  OutScaling=2^0
  Delay2 : xbsIndex_r4/Delay  en=off  latency=1  dbl_ovrd=off  reg_retiming=off  block_type=delay
      settings: infoedit="Delay line having  configurable length.<P><P>Hardware notes: A delay line is a chain, each link of which is an SRL16 followed by a flip-flop. If register retiming is enabled, the delay line is a chain of flip-flops."  xl_area=[0, 0, 0, 0, 0, 0, 0]  block_version=VER_STRING_GOES_HERE
  Delay3 : xbsIndex_r4/Delay  en=off  latency=1  dbl_ovrd=off  reg_retiming=off  block_type=delay
      settings: infoedit="Delay line having  configurable length.<P><P>Hardware notes: A delay line is a chain, each link of which is an SRL16 followed by a flip-flop. If register retiming is enabled, the delay line is a chain of flip-flops."  xl_area=[0, 0, 0, 0, 0, 0, 0]  block_version=VER_STRING_GOES_HERE
  "Interleaver/De-interleaver 6.0 " : xbsIndex_r4/Interleaver//De-interleaver 6.0   memory_style=Automatic  symbol_width=8  sid_type=Forney  mode=Interleaver  symbol_memory=Internal  number_of_branches=12  architecture=ROM_based  number_of_configurations=1  branch_length_constant=17  branch_length_coe_file_name='no_coe_file_loaded'  branch_length_type=constant_difference_between_consecutive_branches  number_of_rows_constant_value=15  row_port_width=4  minimum_rows=15  number_of_rows_selectable_value=4  number_of_rows=constant  number_of_columns_constant_value=15  col_port_width=4  minimum_columns=15  number_of_columns_selectable_value=4  number_of_columns=constant  row_permutations=None  column_permutations=None  coe_file='no_coe_file_loaded'  block_size_constant_value=225  block_size_port_width=8  block_size_type=rows_columns  row_valid=off  block_size_valid=off  ce=off  rfd=off  row_sel_valid=off  block_start=off  sclr=off  rffd=off  col_valid=off  block_end=off  ndo=off  fdo=off  col_sel_valid=off  nd=on  rdy=on  pipelining=minimum  ip_name=Interleaver/De-interleaver  ip_version=6.0  dsptool_ready=true  ipcore_usecache=true  ipcore_useipmodelcache=true  wrapper_available=true  port_translation_map={ 'ce' => 'en', 'sclr' => 'rst'}  structural_sim=false  ipcore_verbose=false  ipcore_do_not_force_period=true  block_type=sid_v6_0
      settings: infoedit=Forney Information : The Forney type is composed of a user-defined number of delay-line shift registers. The length of each of the delay-line shift registers can be specified using a COE file, or by setting the difference in the length of consecutive delay line shift registers to a fixed, user-defined value. <br> Rectangular Information : The Rectangular Block type is composed of a rectangular array of memory elements, where the number of rows and columns in the array is user-defined. The number of rows and columns can be constant or run-time configurable. The elements are written to row-wise, and read out column-wise, or vice versa, depending on which mode is selected. This type supports user-defined inter-row and inter-column permutations. It also supports pruning - cases where the block size is less than the product of the number of rows and columns.  block_version=12.1
  Rising Edge Detector1 : Subsystem
  dout : Outport  OutDataType=sfix(16)  OutScaling=2^0
  vout : Outport  Port=2  OutDataType=sfix(16)  OutScaling=2^0
  wires:
  "Interleaver/De-interleaver 6.0 "/2 -> vout/1
  "Interleaver/De-interleaver 6.0 "/1 -> dout/1
  vin/1 -> Rising Edge Detector1/1(Din), Delay3/1
  din/1 -> Delay2/1
  Delay2/1 -> "Interleaver/De-interleaver 6.0 "/1
  Delay3/1 -> "Interleaver/De-interleaver 6.0 "/2
  Rising Edge Detector1/1(Dout) -> "Interleaver/De-interleaver 6.0 "/3

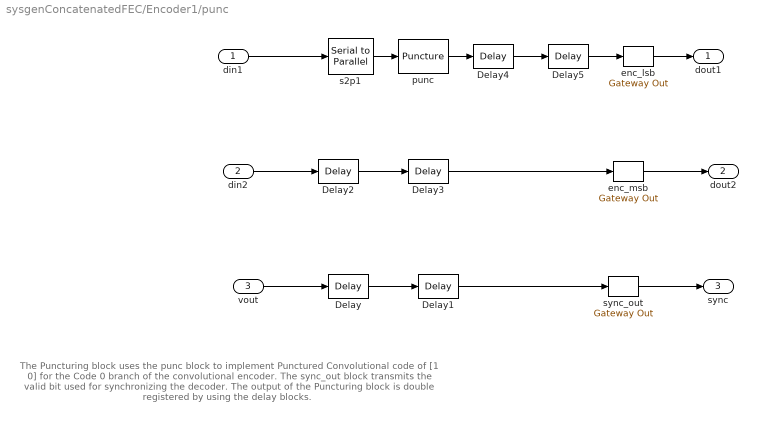
== system sysgenConcatenatedFEC/Encoder1/punc ==
  note: The Puncturing block uses the punc block to implement Punctured Convolutional code of  [1 0] for the Code 0 branch
      | of the convolutional encoder. The sync_out block transmits the valid bit used for synchronizing the decoder.
      |  The output of the Puncturing block is double registered by using the delay blocks.
  din1 : Inport  OutDataType=sfix(16)  OutScaling=2^0
  din2 : Inport  Port=2  OutDataType=sfix(16)  OutScaling=2^0
  vout : Inport  Port=3  OutDataType=sfix(16)  OutScaling=2^0
  Delay{,1..5} (6 alike) : xbsIndex_r4/Delay  en=off  latency=1  dbl_ovrd=off  reg_retiming=off  block_type=delay
      settings: infoedit="Delay line having  configurable length.<P><P>Hardware notes: A delay line is a chain, each link of which is an SRL16 followed by a flip-flop. If register retiming is enabled, the delay line is a chain of flip-flops."  xl_area=[1 1 0 0 0 0 0]  block_version=VER_STRING_GOES_HERE
  enc_lsb : xbsIndex_r4/Gateway Out  hdl_port=on  timing_constraint=None  locs_specified=off  LOCs={}  block_type=gatewayout
      settings: infoedit="Gateway out block.  Converts Xilinx fixed point inputs into ouputs of type Simulink integer, double, or fixed point.<P><P>Hardware notes:  In hardware these blocks become top level output ports or are discarded, depending on how they are configured."  xl_area=[0 0 0 0 1 0 0]  block_version=VER_STRING_GOES_HERE
  enc_msb : xbsIndex_r4/Gateway Out  hdl_port=on  timing_constraint=None  locs_specified=off  LOCs={}  block_type=gatewayout
      settings: infoedit="Gateway out block.  Converts Xilinx fixed point inputs into ouputs of type Simulink integer, double, or fixed point.<P><P>Hardware notes:  In hardware these blocks become top level output ports or are discarded, depending on how they are configured."  xl_area=[0 0 0 0 1 0 0]  block_version=VER_STRING_GOES_HERE
  punc : xbsIndex_r4/Puncture  punc_char=[1 0]  dbl_ovrd=off  block_type=puncture
      settings: infoedit=Reads values from the input port, removes the bits corresponding to zeros in the puncture code, then presents the remaining bits at the output port.<P><P>Hardware notes: In hardware this block costs nothing.  block_version=VER_STRING_GOES_HERE
  s2p1 : xbsIndex_r4/Serial to Parallel  input_order=Least Significant Word First  arith_type=Unsigned  output_bits=2  bin_pt=0  en=off  latency=1  dbl_ovrd=off  block_type=s2p
      settings: infoedit=Groups of samples presented serially at the input become single samples presented at the output.  xl_area=[2 3 0 0 0 0 0]  block_version=VER_STRING_GOES_HERE
  sync_out : xbsIndex_r4/Gateway Out  hdl_port=on  timing_constraint=None  locs_specified=off  LOCs={}  block_type=gatewayout
      settings: infoedit="Gateway out block.  Converts Xilinx fixed point inputs into ouputs of type Simulink integer, double, or fixed point.<P><P>Hardware notes:  In hardware these blocks become top level output ports or are discarded, depending on how they are configured."  xl_area=[0 0 0 0 1 0 0]  block_version=VER_STRING_GOES_HERE
  dout1 : Outport  OutDataType=sfix(16)  OutScaling=2^0
  dout2 : Outport  Port=2  OutDataType=sfix(16)  OutScaling=2^0
  sync : Outport  Port=3  OutDataType=sfix(16)  OutScaling=2^0
  wires:
  din2/1 -> Delay2/1
  vout/1 -> Delay/1
  punc/1 -> Delay4/1
  Delay5/1 -> enc_lsb/1
  Delay4/1 -> Delay5/1
  Delay3/1 -> enc_msb/1
  Delay2/1 -> Delay3/1
  Delay1/1 -> sync_out/1
  Delay/1 -> Delay1/1
  din1/1 -> s2p1/1
  s2p1/1 -> punc/1
  sync_out/1 -> sync/1
  enc_msb/1 -> dout2/1
  enc_lsb/1 -> dout1/1
